simulink model "masa_resorte_amortiguador"  (R2016a)
settings: Solver=ode1  StartTime=0.0  StopTime=10.0  FixedStep=1e-3  RelTol=1e-3
settings Model: Creator=Facundo Mosquera  LastModifiedBy=Facundo Mosquera

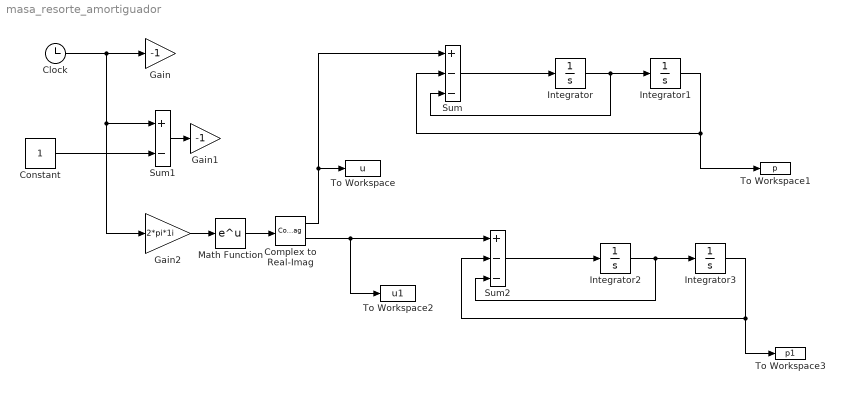
== system masa_resorte_amortiguador ==
  Clock : Clock
  Complex to Real-Imag : ComplexToRealImag
  Constant : Constant
  Gain : Gain  Gain=-1
  Gain1 : Gain  Gain=-1
  Gain2 : Gain  Gain=2*pi*1i
  Integrator{,1..3} (4 alike) : Integrator
  Math Function : Math  SaturateOnIntegerOverflow=on
  Sum : Sum  Inputs=+--
  Sum1 : Sum  Inputs=+-
  Sum2 : Sum  Inputs=+--
  To Workspace : ToWorkspace  VariableName=u  SampleTime=-1
  To Workspace1 : ToWorkspace  VariableName=p  SampleTime=-1
  To Workspace2 : ToWorkspace  VariableName=u1  SampleTime=-1
  To Workspace3 : ToWorkspace  VariableName=p1  SampleTime=-1
  wires:
  Integrator/1 -> Sum/3, Integrator1/1
  Integrator1/1 -> To Workspace1/1, Sum/2
  Sum/1 -> Integrator/1
  Clock/1 -> Gain2/1, Sum1/1, Gain/1
  Sum1/1 -> Gain1/1
  Constant/1 -> Sum1/2
  Complex to Real-Imag/1 -> Sum/1, To Workspace/1
  Integrator2/1 -> Sum2/3, Integrator3/1
  Integrator3/1 -> To Workspace3/1, Sum2/2
  Sum2/1 -> Integrator2/1
  Complex to Real-Imag/2 -> To Workspace2/1, Sum2/1
  Gain2/1 -> Math Function/1
  Math Function/1 -> Complex to Real-Imag/1
